simulink model "PackSony18650"  (R2019b)
settings: Solver=VariableStepAuto  StartTime=0.0  StopTime=10.0  RelTol=1e-3
model workspace (MAT data in the model file):
  BattCapinit = 2.85
  BattTempBp = [-10 0 10 25 40 45]
  CapLUTBp = [0 5 10 20 30 40 50 60 70 80 90 100]
  CapNom = [2.51789473684 2.65254736842 3.12 3.12]
  CapSOCBp = [0 5 10 20 30 40 50 60 70 80 90 100]
  CapTem = [-10 0 23 45]
  Em = [3 3.45 3.68 3.74 3.77 3.79 3.82 3.87 3.92 3.98 4.06 4.2]
  Np = 5
  Ns = 112
  RInt = [18  17  16  15  13  11  10  9.5  9.5  9.5  9.5  9.5; 18  16  15  13  11  10  9.5  9  9  9  9  9; 18  15  13  11  10  9  8.5  8.5  8.5  8.5  8.5  8.5; 18  9  8  8  8  8  8  8  8  8  8  8; 18  8  8  8  8  8  8  8  8  8  8  8; 18  8  8  8  8  8  8  8  8  8  8  8]
settings Model: OrderedModelArguments=off  Creator=ZHOU Jinhan  LastModifiedBy=ZHOU Jinhan

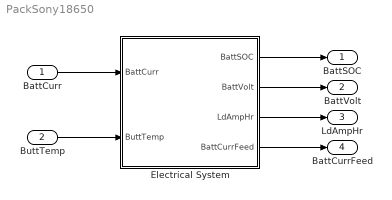
== system PackSony18650 ==
  BattCurr : Inport
  ButtTemp : Inport  Port=2
  Electrical System : Subsystem  mask{RInt=[18 17 16 15 13 11 10 9.5 9.5 9.5 9.5 9.5;18 16 15 13 11 10 9.5 9 9 9 9 9;18 15 13 11 10 9 8.5 8.5 8.5 8.5 8.5 8.5;18 9 8 8 8 8 8 8 8 8 8 8;18 8 8 8 8 8 8 8 8 8 8 8;18 8 8 8 8 8 8 8 8 8 8 8], BattCapinit=2.85, CapLUTBp=[0 5 10 20 30 40 50 60 70 80 90 100], CapSOCBp=[0 5 10 20 30 40 50 60 70 80 90 100], BattTempBp=[-10 0 10 25 40 45], Em=[3 3.45 3.68 3.74 3.77 3.79 3.82 3.87 3.92 3.98 4.06 4.2], Np=5, Ns=112, CapTem=[-10 0 23 45], CapNom=[2.517894736842106 2.652547368421053 3.120000000000001 3.120000000000001]}
      mask Display: image('$imagefile'); % Use "Edit Image" on toolstrip to change.
  BattSOC : Outport
  BattVolt : Outport  Port=2
  LdAmpHr : Outport  Port=3
  BattCurrFeed : Outport  Port=4
  wires:
  BattCurr/1 -> Electrical System/1(BattCurr)
  ButtTemp/1 -> Electrical System/2(ButtTemp)
  Electrical System/1(BattSOC) -> BattSOC/1
  Electrical System/2(BattVolt) -> BattVolt/1
  Electrical System/3(LdAmpHr) -> LdAmpHr/1
  Electrical System/4(BattCurrFeed) -> BattCurrFeed/1

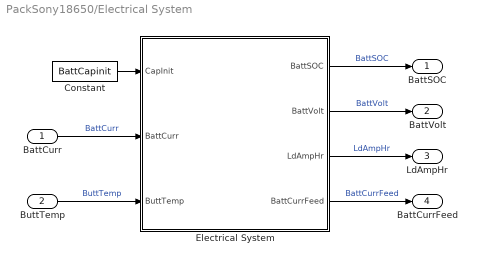
== system PackSony18650/Electrical System ==
  BattCurr : Inport
  ButtTemp : Inport  Port=2
  Constant : Constant  Value=BattCapinit
  Electrical System : Subsystem
  BattSOC : Outport
  BattVolt : Outport  Port=2
  LdAmpHr : Outport  Port=3
  BattCurrFeed : Outport  Port=4
  wires:
  Constant/1 -> Electrical System/1(CapInit)
  Electrical System/2(BattVolt) -> BattVolt/1  "BattVolt"
  BattCurr/1 -> Electrical System/2(BattCurr)  "BattCurr"
  Electrical System/3(LdAmpHr) -> LdAmpHr/1  "LdAmpHr"
  Electrical System/1(BattSOC) -> BattSOC/1  "BattSOC"
  Electrical System/4(BattCurrFeed) -> BattCurrFeed/1  "BattCurrFeed"
  ButtTemp/1 -> Electrical System/3(ButtTemp)  "ButtTemp"

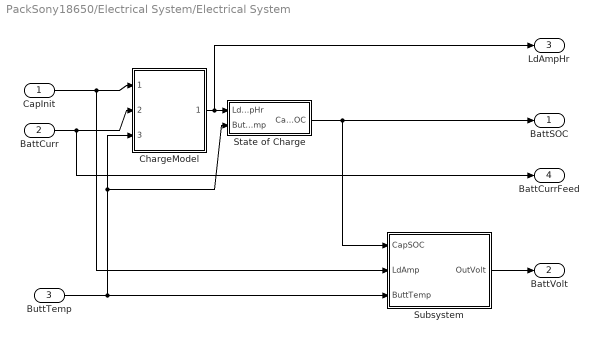
== system PackSony18650/Electrical System/Electrical System ==
  CapInit : Inport
  BattCurr : Inport  Port=2
  ButtTemp : Inport  Port=3
  ChargeModel : Subsystem
  State of Charge : Subsystem
  Subsystem : Subsystem
  BattSOC : Outport
  BattVolt : Outport  Port=2
  LdAmpHr : Outport  Port=3
  BattCurrFeed : Outport  Port=4
  wires:
  ChargeModel/1(LdAmpHr) -> LdAmpHr/1, State of Charge/1(LdAmpHr)
  State of Charge/1(CapSOC) -> BattSOC/1, Subsystem/1(CapSOC)
  CapInit/1 -> Subsystem/2(LdAmp), ChargeModel/1(CapInit)
  BattCurr/1 -> BattCurrFeed/1, ChargeModel/2(BattCurr)
  Subsystem/1(OutVolt) -> BattVolt/1
  ButtTemp/1 -> State of Charge/2(ButtTemp), ChargeModel/3(ButtTemp), Subsystem/3(ButtTemp)

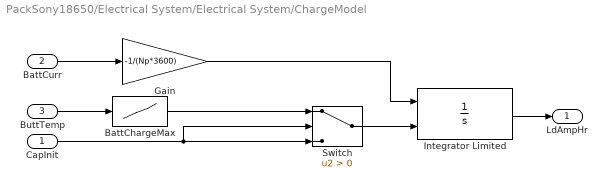
== system PackSony18650/Electrical System/Electrical System/ChargeModel ==
  CapInit : Inport
  BattCurr : Inport  Port=2
  ButtTemp : Inport  Port=3
  BattChargeMax : Lookup_n-D  NumberOfTableDimensions=1  BreakpointsForDimension1=CapTem  Table=CapNom  InterpMethod=Linear Lagrange  InternalRulePriority=Speed  RndMeth=Simplest  InputSameDT=on
  Gain : Gain  Gain=-1/(Np*3600)
  Integrator Limited : Integrator  InitialConditionSource=external  LimitOutput=on  UpperSaturationLimit=1  LowerSaturationLimit=0
  Switch : Switch  Criteria=u2 > Threshold
  LdAmpHr : Outport
  wires:
  BattChargeMax/1 -> Switch/1
  BattCurr/1 -> Gain/1
  Gain/1 -> Integrator Limited/1
  CapInit/1 -> Switch/2, Switch/3
  Integrator Limited/1 -> LdAmpHr/1
  Switch/1 -> Integrator Limited/2
  ButtTemp/1 -> BattChargeMax/1

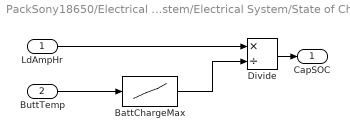
== system PackSony18650/Electrical System/Electrical System/State of Charge ==
  LdAmpHr : Inport
  ButtTemp : Inport  Port=2
  BattChargeMax : Lookup_n-D  NumberOfTableDimensions=1  BreakpointsForDimension1=CapTem  Table=CapNom  InterpMethod=Linear Lagrange  InternalRulePriority=Speed  RndMeth=Simplest  InputSameDT=on
  Divide : Product  Inputs=*/
  CapSOC : Outport
  wires:
  BattChargeMax/1 -> Divide/2
  LdAmpHr/1 -> Divide/1
  Divide/1 -> CapSOC/1
  ButtTemp/1 -> BattChargeMax/1

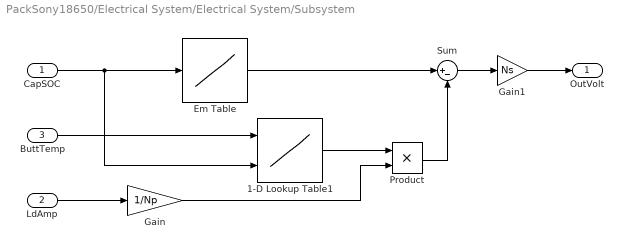
== system PackSony18650/Electrical System/Electrical System/Subsystem ==
  CapSOC : Inport
  LdAmp : Inport  Port=2
  ButtTemp : Inport  Port=3
  1-D Lookup Table1 : Lookup_n-D  BreakpointsForDimension1=BattTempBp  BreakpointsForDimension2=CapSOCBp  Table=RInt.*1e-3  InternalRulePriority=Speed  RndMeth=Simplest  InputSameDT=on
  Em Table : Lookup_n-D  NumberOfTableDimensions=1  BreakpointsForDimension1=CapLUTBp  Table=Em  InterpMethod=Linear Lagrange  InternalRulePriority=Speed  RndMeth=Simplest  InputSameDT=on
  Gain : Gain  Gain=1/Np
  Gain1 : Gain  Gain=Ns
  Product : Product
  Sum : Sum  Inputs=|+-
  OutVolt : Outport
  wires:
  ButtTemp/1 -> 1-D Lookup Table1/1
  Em Table/1 -> Sum/1
  Sum/1 -> Gain1/1
  Gain/1 -> Product/2
  Product/1 -> Sum/2
  LdAmp/1 -> Gain/1
  CapSOC/1 -> 1-D Lookup Table1/2, Em Table/1
  Gain1/1 -> OutVolt/1
  1-D Lookup Table1/1 -> Product/1
